simulink model "vrmaglev_rtwin"  (Simulink 6.0)
settings: Solver=ode5  SolverMode=SingleTasking  StartTime=0.0  StopTime=Inf  FixedStep=1e-3  MaxStep=0.001  RelTol=1e-3  AbsTol=1e-5
PreLoadFcn:
  | Ts=1e-3;
PostLoadFcn:
  | if ~exist('dsparch4','file') errordlg('Signal Processing Blockset is required to run this demo.', 'Signal Processing Blockset required'); end
undefined symbols (not defined in the file or in its folder): Humusoft, MF614
libraries: simulink x3, rtwinlib x2, vrlib x2, dsparch4 x1
settings Model: CovMetricSettings=d  Creator=Sehnal  LastModifiedBy=Sehnal  ExtModeTrigDuration=5000  ExtModeTrigLevel=0.500000  BufferReuse=off  UpdateModelReferenceTargets=IfOutOfDate
settings ConfigSet: SimulationMode=external
settings DataIOCC: SaveOutput=off  SaveTime=off  SignalLoggingName=logsOut
settings OptimizationCC: BlockReduction=off  BooleanDataType=off  OptimizeBlockIOStorage=off  BufferReuse=off  ExpressionFolding=off  LocalBlockOutputs=off
settings DebuggingCC: CheckExecutionContextPreStartOutputMsg=on  CheckExecutionContextRuntimeOutputMsg=on  SolverPrmCheckMsg=none
settings HardwareCC: TargetUnknown=on
settings ModelReferenceCC: UpdateModelReferenceTargets=IfOutOfDate
settings RTWCC: SystemTargetFile=rtwin.tlc  TemplateMakefile=rtwin.tmf  RetainRTWFile=on  ProcessScript=rtwin_make_rtw_hook
settings RTWinTargetCC: TargetFcnLib=ansi_tfl_tmw.mat  GenFloatMathFcnCalls=ANSI_C  UtilityFuncGeneration=Automatic  ModelReferenceCompliant=off  MatFileLogging=on  LifeSpan=inf  CCOptimize=on
settings SFSimCC: SFSimApplyToAllLibs=on  SFSimBuildMode=Incremental

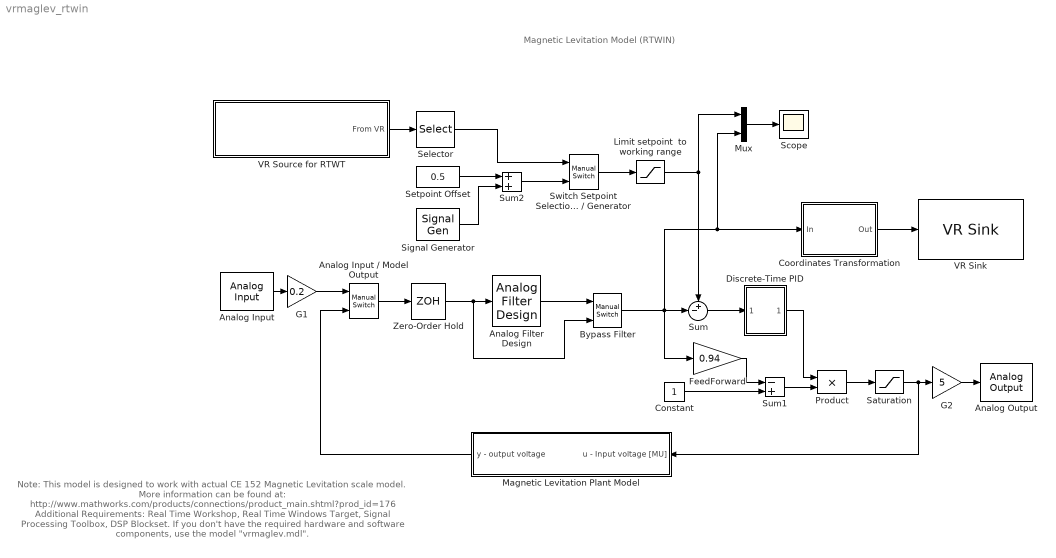
== system vrmaglev_rtwin ==
  note: Magnetic Levitation Model
      | (RTWIN)
  note: Note:
      | This model is designed to work with actual CE 152 Magnetic Levitation scale model. More information can be found at:
      | http://www.mathworks.com/products/connections/product_main.shtml?prod_id=176
      | Additional Requirements: Real Time Workshop, Real Time Windows Target, Signal Processing Toolbox, DSP Blockset.
      | If you don't have the required hardware and software components, use the model "vrmaglev.mdl".
  Analog Filter Design : dsparch4/Analog Filter Design  method=Butterworth  filttype=Lowpass  N=2  Wlo=2*pi*100  Whi=80  Rp=2  Rs=40
  Analog Input : rtwinlib/Analog Input  SampleTime=1e-3  DrvName=Humusoft/MF614  DrvAddress=4294967295  DrvOptions=0  Channels=1  RangeMode=1  VoltRange=2
      settings: AttributesFormatString=Humusoft\nMF614 [auto]
  "Analog Input / Model Output " : simulink/Signal Routing/Manual Switch  sw=1  action=0
  Analog Output : rtwinlib/Analog Output  SampleTime=1e-3  DrvName=Humusoft/MF614  DrvAddress=4294967295  DrvOptions=0  Channels=1  RangeMode=1  VoltRange=1  InitialValue=0  FinalValue=0
      settings: AttributesFormatString=Humusoft\nMF614 [auto]
  Bypass Filter : simulink/Signal Routing/Manual Switch  sw=1  action=0
  Constant : Constant
  Coordinates Transformation : Subsystem  EnableExecutionContextPropagation=on
  Discrete-Time PID : Subsystem  EnableExecutionContextPropagation=on  mask(PID){Kp=1, Ki=10, Kd=0.03, Ts=Ts}
      mask prompts: Ts "Sample time:"
      mask help: Discrete-time PID controller with limited integrator
      mask Display: disp('PID');
  FeedForward : Gain  Gain=0.94  SaturateOnIntegerOverflow=on
  G1 : Gain  Gain=0.2  SaturateOnIntegerOverflow=on
  G2 : Gain  Gain=5  SaturateOnIntegerOverflow=on
  "Limit setpoint  to working range  " : Saturate  UpperLimit=0.8  LowerLimit=0  ZeroCross=off
  Magnetic Levitation Plant Model : Subsystem  Orientation=left  EnableExecutionContextPropagation=on
  Mux : Mux  Inputs=2
  Product : Product  SaturateOnIntegerOverflow=on  InputSameDT=on
  Saturation : Saturate  UpperLimit=1  LowerLimit=0  ZeroCross=off
  Scope : Scope
      settings: TimeRange=5  YMin=-0.0227122  YMax=1.027  DataFormat=Structure  MaxDataPoints=250  SampleInput=on  SampleTime=0.02
  Selector : Selector  Elements=[2]  InputPortWidth=3
  Setpoint Offset : Constant  Value=0.5
  Signal Generator : SignalGenerator  WaveForm=square  Amplitude=0.2  Frequency=5.0  Units=rad/sec
  Sum : Sum  Inputs=+-|  SaturateOnIntegerOverflow=on  InputSameDT=on
  Sum1 : Sum  Inputs=-+  SaturateOnIntegerOverflow=on  InputSameDT=on
  Sum2 : Sum  SaturateOnIntegerOverflow=on  InputSameDT=on
  Switch Setpoint Selection Method Virtual Reality / Generator : simulink/Signal Routing/Manual Switch  sw=0  action=0
  VR Sink : vrlib/VR Sink  SampleTime=0.1  ViewEnable=on  RemoteChange=off  RemoteView=off  FieldsWritten=Ball.translation.3.1.double  WorldFileName=maglev.wrl  AutoView=on
  VR Source for RTWT : Subsystem  EnableExecutionContextPropagation=on  mask(VR Source for RTWT){Ts=0.2, vr_world='maglev.wrl', vr_field='Grab_Sensor.translation_changed'}
      mask prompts: Ts "Sample time:"; vr_world "VRML world name:"; vr_field "VRML Node.Field name:"
      mask Display: image(imread('vrblockicon.png')); port_label('output', 1, vr_field);
  Zero-Order Hold : ZeroOrderHold  SampleTime=Ts
  wires:
  Constant/1 -> Sum1/2
  Sum1/1 -> Product/2
  FeedForward/1 -> Sum1/1
  Sum2/1 -> Switch Setpoint Selection Method Virtual Reality / Generator/2
  Sum/1 -> Discrete-Time PID/1(in_1)
  Discrete-Time PID/1(out_1) -> Product/1
  Signal Generator/1 -> Sum2/2
  Setpoint Offset/1 -> Sum2/1
  Switch Setpoint Selection Method Virtual Reality / Generator/1 -> "Limit setpoint  to working range  "/1
  Mux/1 -> Scope/1
  Product/1 -> Saturation/1
  Analog Input/1 -> G1/1
  "Analog Input / Model Output "/1 -> Zero-Order Hold/1
  Saturation/1 -> Magnetic Levitation Plant Model/1(u - Input voltage [MU]), G2/1
  Magnetic Levitation Plant Model/1(y - output voltage) -> "Analog Input / Model Output "/2
  Coordinates Transformation/1(Out) -> VR Sink/1
  G1/1 -> "Analog Input / Model Output "/1
  G2/1 -> Analog Output/1
  Analog Filter Design/1 -> Bypass Filter/1
  VR Source for RTWT/1(From VR) -> Selector/1
  Selector/1 -> Switch Setpoint Selection Method Virtual Reality / Generator/1
  "Limit setpoint  to working range  "/1 -> Sum/1, Mux/1
  Bypass Filter/1 -> Sum/2, FeedForward/1, Coordinates Transformation/1(In), Mux/2
  Zero-Order Hold/1 -> Analog Filter Design/1, Bypass Filter/2

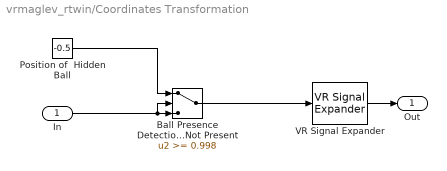
== system vrmaglev_rtwin/Coordinates Transformation ==
  In : Inport  LatchInput=off
  Ball Presence Detection Value > Threshold = Ball Not Present : Switch  Threshold=0.998  InputSameDT=on
  Position of  Hidden Ball : Constant  Value=-0.5
  VR Signal Expander : vrlib/VR Signal Expander  outwidth=3  outidx=[2]
  Out : Outport
  wires:
  Position of  Hidden Ball/1 -> Ball Presence Detection Value > Threshold = Ball Not Present/1
  Ball Presence Detection Value > Threshold = Ball Not Present/1 -> VR Signal Expander/1
  VR Signal Expander/1 -> Out/1
  In/1 -> Ball Presence Detection Value > Threshold = Ball Not Present/3, Ball Presence Detection Value > Threshold = Ball Not Present/2

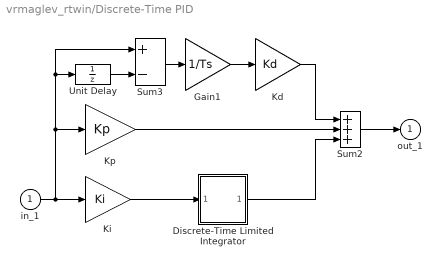
== system vrmaglev_rtwin/Discrete-Time PID ==
  in_1 : Inport  LatchInput=off
  Discrete-Time Limited Integrator : Subsystem  EnableExecutionContextPropagation=on  mask(Discrete-Time Limited Integrator.){@1=0, @2=2, @3=0, @4=Ts}
      mask prompts: @1 "Lower bound:"; @2 "Upper bound:"; @3 "Initial condition:"; @4 "Sampling Time:"
      mask help: Discrete-Time Limited Integrator.
      mask init:
      | lower_limit=@1;upper_limit=@2;X0=@3;Ts=@4;
      mask Help: Discrete-Time Limited Integrator. Unmask to see details.
      mask Display: plot(-1,-0.2,3.5,1.2,[0,1,2,2.9],[0,0,1,1],[0,1],[0.5,0.5], [.5,.5], [.8,.6], [.05,.35,.05,.35],[.4,.4,.2,.2], [.45,.65],[.3,.3], [.9,.9],[.2,.4]);
  Gain1 : Gain  Gain=1/Ts  SaturateOnIntegerOverflow=on
  Kd : Gain  Gain=Kd  SaturateOnIntegerOverflow=on
  Ki : Gain  Gain=Ki  SaturateOnIntegerOverflow=on
  Kp : Gain  Gain=Kp  SaturateOnIntegerOverflow=on
  Sum2 : Sum  Inputs=+++  SaturateOnIntegerOverflow=on  InputSameDT=on
  Sum3 : Sum  Inputs=+-  SaturateOnIntegerOverflow=on  InputSameDT=on
  Unit Delay : UnitDelay  SampleTime=Ts
  out_1 : Outport  InitialOutput=0
  wires:
  Unit Delay/1 -> Sum3/2
  Kd/1 -> Sum2/1
  Kp/1 -> Sum2/2
  Sum2/1 -> out_1/1
  Sum3/1 -> Gain1/1
  Gain1/1 -> Kd/1
  in_1/1 -> Ki/1, Sum3/1, Unit Delay/1, Kp/1
  Ki/1 -> Discrete-Time Limited Integrator/1(in_1)
  Discrete-Time Limited Integrator/1(out_1) -> Sum2/3

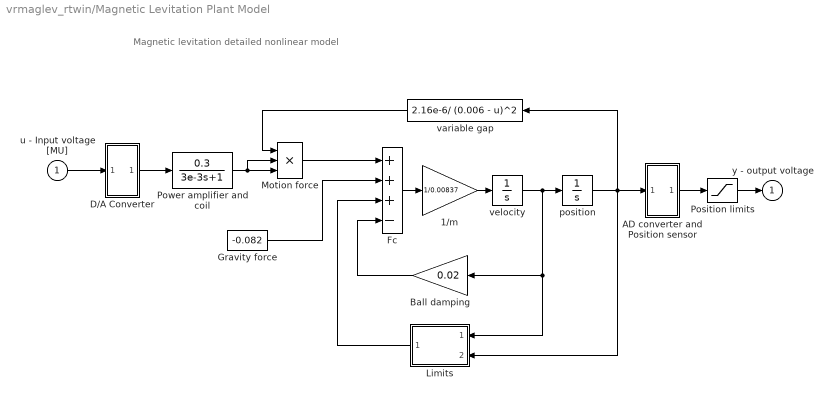
== system vrmaglev_rtwin/Magnetic Levitation Plant Model ==
  note: Magnetic levitation
      | detailed nonlinear model
  u - Input voltage [MU] : Inport  LatchInput=off
  1/m : Gain  Gain=1/0.00837  SaturateOnIntegerOverflow=on
  AD converter and Position sensor : Subsystem  EnableExecutionContextPropagation=on
      mask Display: disp('A/D')
  Ball damping : Gain  Orientation=left  Gain=0.02  SaturateOnIntegerOverflow=on
  D/A Converter : Subsystem  EnableExecutionContextPropagation=on
      mask Display: disp('D/A')
  Fc : Sum  Inputs=+++-  SaturateOnIntegerOverflow=on  InputSameDT=on
  Gravity force : Constant  Value=-0.082
  Limits : Subsystem  Orientation=left  EnableExecutionContextPropagation=on
      mask Display: disp('LIMIT')
  Motion force : Product  Inputs=3  SaturateOnIntegerOverflow=on  InputSameDT=on
  Position limits : Saturate  UpperLimit=0.998  LowerLimit=0  ZeroCross=off
  Power amplifier and coil : TransferFcn  Numerator=[0.3]  Denominator=[3e-3 1]
  position : Integrator  LimitOutput=on  UpperSaturationLimit=0.005  LowerSaturationLimit=0  ZeroCross=off
  variable gap : Fcn  Orientation=left  Expr=2.16e-6/ (0.006 - u)^2
  velocity : Integrator  UpperSaturationLimit=Inf  LowerSaturationLimit=-Inf  ZeroCross=off
  y - output voltage : Outport
  wires:
  velocity/1 -> Ball damping/1, Limits/1(velocity), position/1
  Ball damping/1 -> Fc/4
  variable gap/1 -> Motion force/1
  1/m/1 -> velocity/1
  Fc/1 -> 1/m/1
  Motion force/1 -> Fc/1
  Gravity force/1 -> Fc/2
  D/A Converter/1(out_1) -> Power amplifier and coil/1
  u - Input voltage [MU]/1 -> D/A Converter/1(in_1)
  AD converter and Position sensor/1(out_1) -> Position limits/1
  position/1 -> Limits/2(position), variable gap/1, AD converter and Position sensor/1(in_1)
  Limits/1(force) -> Fc/3
  Power amplifier and coil/1 -> Motion force/3, Motion force/2
  Position limits/1 -> y - output voltage/1

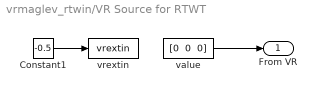
== system vrmaglev_rtwin/VR Source for RTWT ==
  Constant1 : Constant  Value=-0.5
  value : Constant  Value="[0  0  0]"
  vrextin : S-Function  FunctionName=vrextin  Parameters=Ts, 'maglev.wrl', 'Grab_Sensor.translation_changed'
  From VR : Outport
  wires:
  value/1 -> From VR/1
  Constant1/1 -> vrextin/1

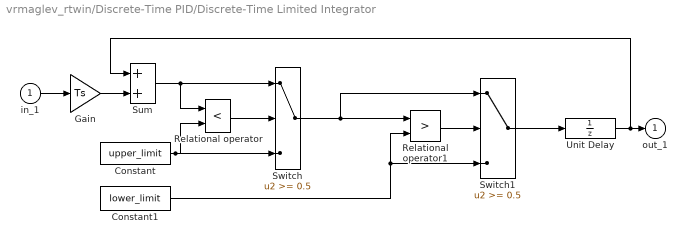
== system vrmaglev_rtwin/Discrete-Time PID/Discrete-Time Limited Integrator ==
  in_1 : Inport  LatchInput=off
  Constant : Constant  Value=upper_limit
  Constant1 : Constant  Value=lower_limit
  Gain : Gain  Gain=Ts  SaturateOnIntegerOverflow=on
  Relational operator : RelationalOperator  Operator=<  InputSameDT=on
  Relational operator1 : RelationalOperator  Operator=>  InputSameDT=on
  Sum : Sum  SaturateOnIntegerOverflow=on  InputSameDT=on
  Switch : Switch  Threshold=0.5  InputSameDT=on
  Switch1 : Switch  Threshold=0.5  InputSameDT=on
  Unit Delay : UnitDelay  X0=X0  SampleTime=Ts
  out_1 : Outport  InitialOutput=0
  wires:
  Unit Delay/1 -> out_1/1, Sum/1
  Switch1/1 -> Unit Delay/1
  Constant1/1 -> Relational operator1/2, Switch1/3
  Relational operator1/1 -> Switch1/2
  Switch/1 -> Relational operator1/1, Switch1/1
  Constant/1 -> Switch/3, Relational operator/2
  Gain/1 -> Sum/2
  Sum/1 -> Switch/1, Relational operator/1
  Relational operator/1 -> Switch/2
  in_1/1 -> Gain/1

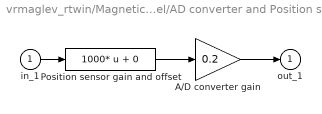
== system vrmaglev_rtwin/Magnetic Levitation Plant Model/AD converter and Position sensor ==
  in_1 : Inport  LatchInput=off
  A/D converter gain : Gain  Gain=0.2  SaturateOnIntegerOverflow=on
  Position sensor gain and offset : Fcn  Expr=1000* u + 0
  out_1 : Outport
  wires:
  in_1/1 -> Position sensor gain and offset/1
  Position sensor gain and offset/1 -> A/D converter gain/1
  A/D converter gain/1 -> out_1/1

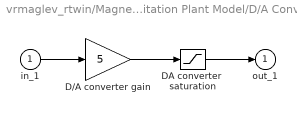
== system vrmaglev_rtwin/Magnetic Levitation Plant Model/D/A Converter ==
  in_1 : Inport  LatchInput=off
  D/A converter gain : Gain  Gain=5  SaturateOnIntegerOverflow=on
  DA converter  saturation : Saturate  UpperLimit=5  LowerLimit=-5  ZeroCross=off
  out_1 : Outport
  wires:
  in_1/1 -> D/A converter gain/1
  DA converter  saturation/1 -> out_1/1
  D/A converter gain/1 -> DA converter  saturation/1

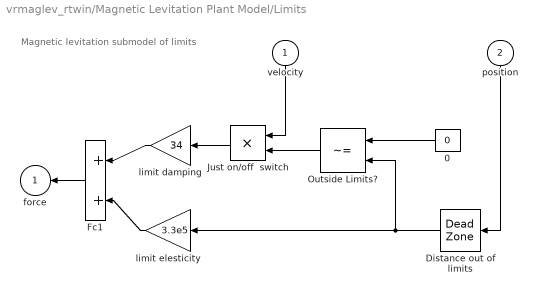
== system vrmaglev_rtwin/Magnetic Levitation Plant Model/Limits ==
  note: Magnetic levitation
      | submodel of limits
  velocity : Inport  Orientation=down  LatchInput=off
  position : Inport  Orientation=down  Port=2  LatchInput=off
  0 : Constant  Orientation=left  Value=0
  Distance out of limits : DeadZone  Orientation=left  LowerValue=0  UpperValue=0.005  ZeroCross=off  SaturateOnIntegerOverflow=on
  Fc1 : Sum  Orientation=left  SaturateOnIntegerOverflow=on  InputSameDT=on
  "Just on/off  switch " : Product  Orientation=left  SaturateOnIntegerOverflow=on  InputSameDT=on
  Outside Limits? : RelationalOperator  Orientation=left  Operator=~=  InputSameDT=on
  limit damping : Gain  Orientation=left  Gain=34  SaturateOnIntegerOverflow=on
  limit elesticity : Gain  Orientation=left  Gain=3.3e5  SaturateOnIntegerOverflow=on
  force : Outport  Orientation=left
  wires:
  Distance out of limits/1 -> Outside Limits?/2, limit elesticity/1
  limit damping/1 -> Fc1/1
  limit elesticity/1 -> Fc1/2
  Outside Limits?/1 -> "Just on/off  switch "/2
  0/1 -> Outside Limits?/1
  "Just on/off  switch "/1 -> limit damping/1
  velocity/1 -> "Just on/off  switch "/1
  Fc1/1 -> force/1
  position/1 -> Distance out of limits/1
